simulink subsystem "controlSystem_block"  (R2022b)
settings: Solver=VariableStepAuto  StartTime=0.0  StopTime=10.0  RelTol=1e-3
undefined symbols (not defined in the file): automatic_control_enable, cVect, daVect, deVect, drVect, manual_control_enable, thrustss, vector_control_enable
libraries: aerolibanimutils x1
settings Model: Creator=lasto  LastModifiedBy=lasto

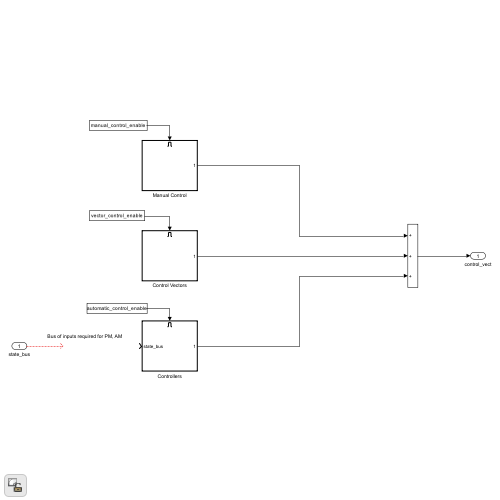
[thumbnail: Simulink's stored preview of the top-level diagram]
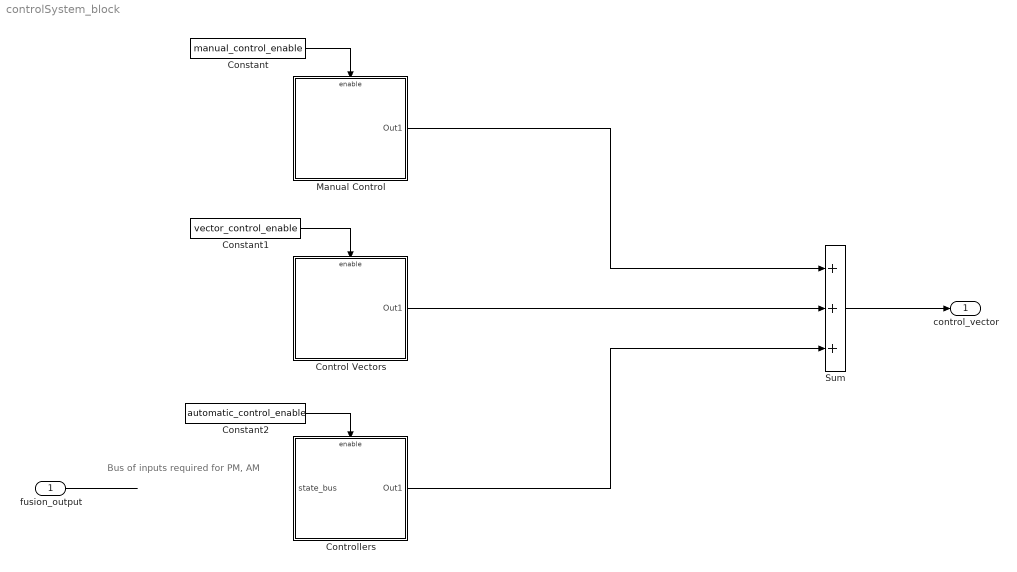
== system controlSystem_block ==
  note: Bus of inputs required for PM, AM
  fusion_output : Inport
  Constant : Constant  Value=manual_control_enable
  Constant1 : Constant  Value=vector_control_enable
  Constant2 : Constant  Value=automatic_control_enable
  Control Vectors : Subsystem
  Controllers : Subsystem
  Manual Control : Subsystem
  Sum : Sum  Inputs=+++
  control_vector : Outport
  wires:
  fusion_output/1 -> ?
  Manual Control/1(Out1) -> Sum/1
  Constant/1 -> Manual Control/Enable
  Control Vectors/1(Out1) -> Sum/2
  Constant1/1 -> Control Vectors/Enable
  Controllers/1(Out1) -> Sum/3
  Constant2/1 -> Controllers/Enable
  Sum/1 -> control_vector/1

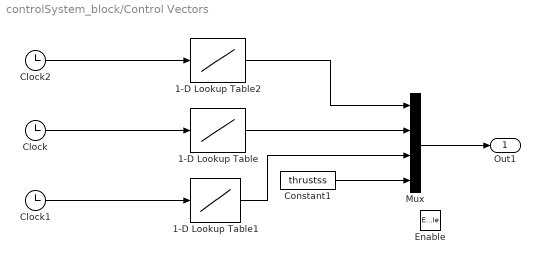
== system controlSystem_block/Control Vectors ==
  Enable : EnablePort
  1-D Lookup Table : Lookup_n-D  NumberOfTableDimensions=1  BreakpointsForDimension1=cVect  Table=deVect  InternalRulePriority=Speed  RndMeth=Simplest
  1-D Lookup Table1 : Lookup_n-D  NumberOfTableDimensions=1  BreakpointsForDimension1=cVect  Table=drVect  InternalRulePriority=Speed  RndMeth=Simplest
  1-D Lookup Table2 : Lookup_n-D  NumberOfTableDimensions=1  BreakpointsForDimension1=cVect  Table=daVect  InternalRulePriority=Speed  RndMeth=Simplest
  Clock : Clock
  Clock1 : Clock
  Clock2 : Clock
  Constant1 : Constant  Value=thrustss
  Mux : Mux
  Out1 : Outport  OutputWhenDisabled=reset  InitialOutput=[0,0,0,0]
  wires:
  Clock2/1 -> 1-D Lookup Table2/1
  Clock1/1 -> 1-D Lookup Table1/1
  Clock/1 -> 1-D Lookup Table/1
  Constant1/1 -> Mux/4
  1-D Lookup Table1/1 -> Mux/3
  1-D Lookup Table2/1 -> Mux/1
  1-D Lookup Table/1 -> Mux/2
  Mux/1 -> Out1/1

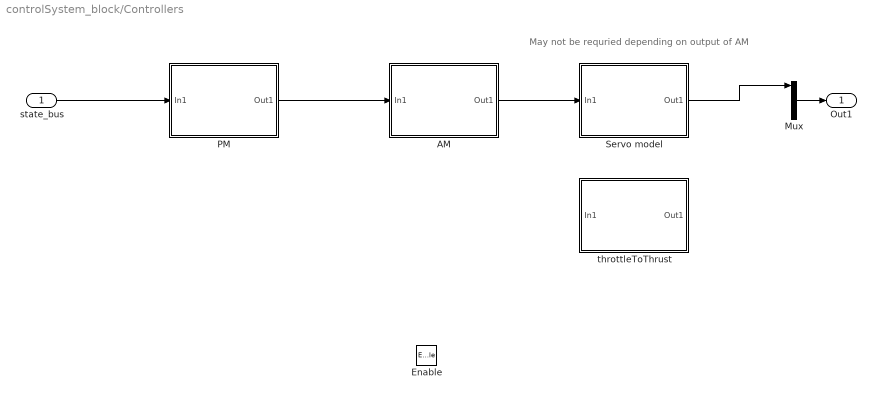
== system controlSystem_block/Controllers ==
  note: May not be requried depending on output of AM
  state_bus : Inport
  Enable : EnablePort
  AM : Subsystem
  Mux : Mux
  PM : Subsystem
  Servo model : Subsystem
  throttleToThrust : Subsystem
  Out1 : Outport  OutputWhenDisabled=reset  InitialOutput=[0,0,0,0]
  wires:
  Mux/1 -> Out1/1
  Servo model/1(Out1) -> Mux/1
  AM/1(Out1) -> Servo model/1(In1)
  PM/1(Out1) -> AM/1(In1)
  state_bus/1 -> PM/1(In1)

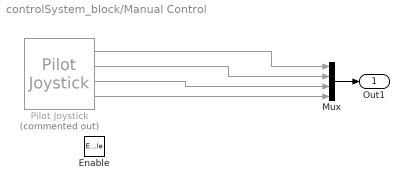
== system controlSystem_block/Manual Control ==
  Enable : EnablePort
  Mux : Mux
  Pilot Joystick : aerolibanimutils/Pilot Joystick  Commented=on  JoystickID=Joystick1  OutputConfiguration=FourAxis  SampleTime=1/30
  Out1 : Outport  OutputWhenDisabled=reset  InitialOutput=[0,0,0,0]
  wires:
  Pilot Joystick/4 -> Mux/4
  Pilot Joystick/3 -> Mux/3
  Pilot Joystick/2 -> Mux/2
  Mux/1 -> Out1/1
  Pilot Joystick/1 -> Mux/1

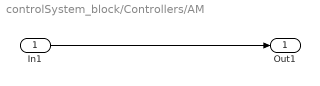
== system controlSystem_block/Controllers/AM ==
  In1 : Inport
  Out1 : Outport
  wires:
  In1/1 -> Out1/1

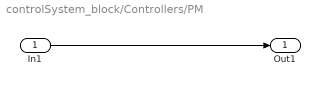
== system controlSystem_block/Controllers/PM ==
  In1 : Inport
  Out1 : Outport
  wires:
  In1/1 -> Out1/1

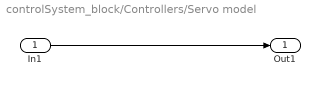
== system controlSystem_block/Controllers/Servo model ==
  In1 : Inport
  Out1 : Outport
  wires:
  In1/1 -> Out1/1

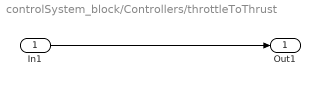
== system controlSystem_block/Controllers/throttleToThrust ==
  In1 : Inport
  Out1 : Outport
  wires:
  In1/1 -> Out1/1
